simulink model "sampleModel27"  (R2021b)
settings: Solver=VariableStepAuto  StartTime=0.0  StopTime=10.0  RelTol=1e-3
undefined symbols (not defined in the file or in its folder): Newton, Raphson
libraries: simulink x5, slpidlib x1
settings Model: Creator=user  LastModifiedBy=user

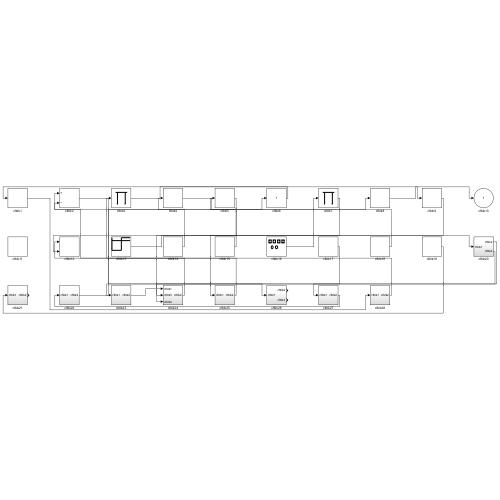
[thumbnail: Simulink's stored preview of the top-level diagram]
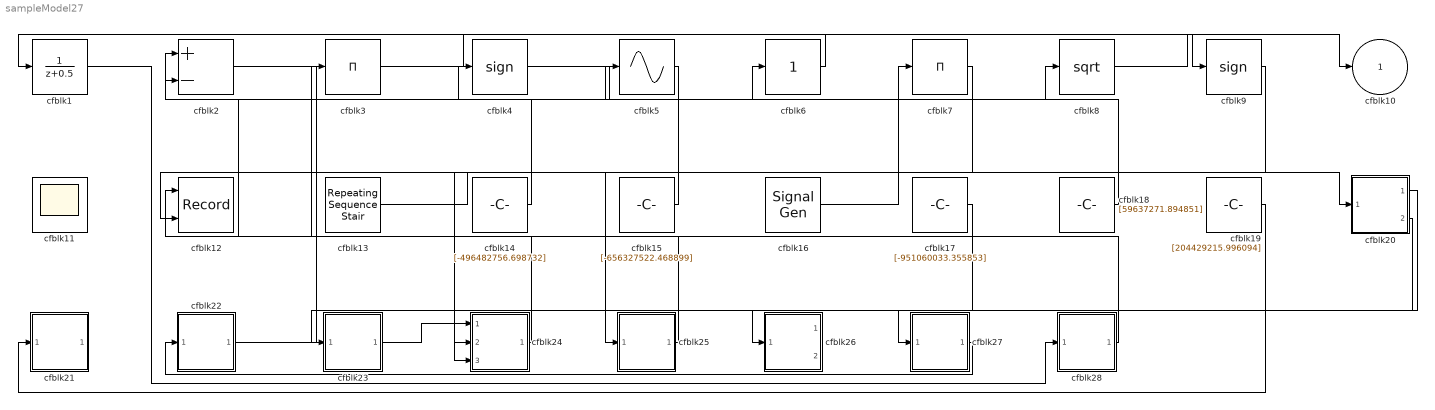
== system sampleModel27 ==
  cfblk1 : DiscreteTransferFcn  SampleTime=1
  cfblk11 : Scope
      settings: Floating=on
  cfblk12 : Record  FileSettingsInternal="{\"entries\":[{\"content\":{\"excelSettings\":{\"content\":{},\"type\":\"Streamout.ExcelSettings\"}},\"type\":\"Streamout.FileSettingStorage\",\"uuid\":\"817101b1-7ee6-489f-8bf2-f4af326754e9\"}],\"packageUris\":[\"http://schema.mathworks.com/mf0/streamout_blocks/R2020a\"],\"version\":\"1.0\"}"  Layout=[1 1]  SignalsInternal="{\"entries\":[{\"content\":{\"signals\":[{\"content\":{\"blockPath\":[\"sampleModel27/cfblk12\"],\"channel\":[],\"dimensions\":[1],\"domain\":\"sampleModel27/cfblk12\",\"lineColor\":\"#a2142f\",\"plots\":[1],\"port\":1,\"sid\":[\"\"],\"signalID\":1067,\"signalName\":\"cfblk24\"},\"type\":\"RecordBlkView.Signal\",\"uuid\":\"11552be4-8ecd-494b-946a-d208da3a0090\"},{\"content\":{\"blockPath\":[\"sampleModel27/cfblk12\"],\"channel\":[],\"dimensions\":[1],\"domain\":\"sampleModel27/cfblk12\",\"lineColor\":\"#139fff\",\"plots\":[1],\"port\":2,\"sid\":[\"\"],\"signalID\":1071,\"signalName\":\"cfblk9\"},\"type\":\"RecordBlkView.Signal\",\"uuid\":\"e2f3f9ab-da11-493e-9bea-993bb7e61e53\"}]},\"type\":\"RecordBlkView.InputSignals\",\"uuid\":\"027c9f95-9f0f-4801-a41c-29daeef56658\"}],\"packageUris\":[\"http://schema.mathworks.com/mf0/streamout_blocks/R2020a\"],\"version\":\"1.0\"}"  VisualizationBindings="{\"xyplotplugin\":{\"info\":[{\"series\":[{\"bindingParametersList\":[{\"parameter\":\"X-Axis\",\"signalID\":1067,\"signalName\":\"cfblk24\"},{\"parameter\":\"Y-Axis\",\"signalID\":1071,\"signalName\":\"cfblk9\"}],\"seriesID\":40632}],\"subplotID\":1}]}}"  CompatibilityTag=XY
  cfblk13 : simulink/Sources/Repeating Sequence Stair  OutValues=[-914274327.688707, 278326402.924223]  tsamp=-1  OutMin=[]  OutMax=[]  OutDataTypeStr=double  OutputDataTypeScalingMode=double  OutDataType=fixdt(0,8)  ConRadixGroup=Best Precision: Vector-wise  OutScaling=2^-12
  cfblk14 : Constant  Value=[-496482756.698732]  SampleTime=1
  cfblk15 : Constant  Value=[-656327522.468899]  SampleTime=1
  cfblk16 : SignalGenerator  Amplitude=[-317971779.391681]
  cfblk17 : Constant  Value=[-951060033.355853]  SampleTime=1
  cfblk18 : Constant  Value=[59637271.894851]  SampleTime=1
  cfblk19 : Constant  Value=[204429215.996094]  SampleTime=1
  cfblk2 : Sum  Inputs=+-
  cfblk20 : Subsystem
  cfblk21 : Subsystem
  cfblk22 : Subsystem
  cfblk23 : Subsystem
  cfblk24 : Subsystem
  cfblk25 : Subsystem
  cfblk26 : Subsystem
  cfblk27 : Subsystem
  cfblk28 : Subsystem
  cfblk3 : Product  Inputs=*
  cfblk4 : Signum
  cfblk5 : Sin  TimeSource=Use external signal  SampleTime=0
  cfblk6 : simulink/Math Operations/Slider Gain  gain=1  low=0  high=2
  cfblk7 : Product  Inputs=*
  cfblk8 : Sqrt  SaturateOnIntegerOverflow=on
  cfblk9 : Signum
  cfblk10 : Outport
  wires:
  cfblk3/1 -> cfblk9/1
  cfblk7/1 -> cfblk25/1(cfblk1)
  cfblk24/1(cfblk2) -> cfblk12/1
  cfblk9/1 -> cfblk12/2
  cfblk2/1 -> cfblk26/1(cfblk1)
  cfblk27/1(cfblk2) -> cfblk22/1(cfblk1)
  cfblk16/1 -> cfblk7/1
  cfblk28/1(cfblk2) -> cfblk3/1
  cfblk17/1 -> cfblk27/1(cfblk1)
  cfblk4/1 -> cfblk6/1
  cfblk1/1 -> cfblk28/1(cfblk1)
  cfblk14/1 -> cfblk2/1
  cfblk6/1 -> cfblk1/1
  cfblk19/1 -> cfblk21/1(cfblk1)
  cfblk15/1 -> cfblk5/1
  cfblk8/1 -> cfblk10/1
  cfblk18/1 -> cfblk4/1
  cfblk23/1(cfblk2) -> cfblk24/1(cfblk1)
  cfblk22/1(cfblk2) -> cfblk8/1
  cfblk13/1 -> cfblk20/1(cfblk1)
  cfblk25/1(cfblk2) -> cfblk2/2
  cfblk5/1 -> cfblk24/2(cfblk3)
  cfblk20/1(cfblk2) -> cfblk23/1(cfblk1)
  cfblk20/2(cfblk4) -> cfblk24/3(cfblk4)

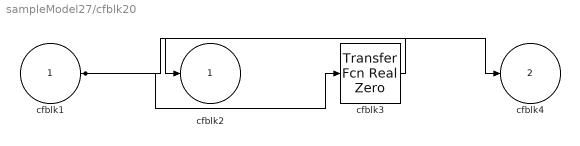
== system sampleModel27/cfblk20 ==
  cfblk1 : Inport
  cfblk3 : simulink/Discrete/Transfer Fcn Real Zero  ZeroZ=0.75  ICPrevInput=0.0  DoSatur=off
      settings: SourceProductBaseCode=SL
  cfblk2 : Outport
  cfblk4 : Outport  Port=2
  wires:
  cfblk3/1 -> cfblk2/1
  cfblk1/1 -> cfblk3/1, cfblk4/1

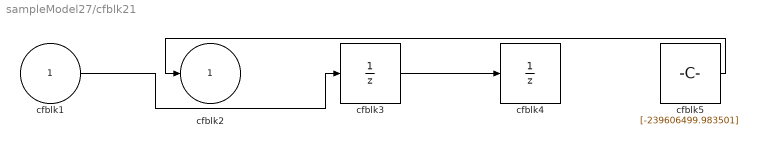
== system sampleModel27/cfblk21 ==
  cfblk1 : Inport
  cfblk3 : UnitDelay  HasFrameUpgradeWarning=on
  cfblk4 : UnitDelay  HasFrameUpgradeWarning=on
  cfblk5 : Constant  Value=[-239606499.983501]  SampleTime=1
  cfblk2 : Outport
  wires:
  cfblk5/1 -> cfblk2/1
  cfblk3/1 -> cfblk4/1
  cfblk1/1 -> cfblk3/1

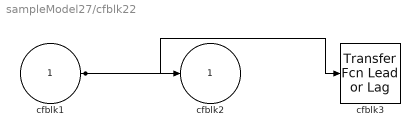
== system sampleModel27/cfblk22 ==
  cfblk1 : Inport
  cfblk3 : simulink/Discrete/Transfer Fcn Lead or Lag  PoleZ=0.95  ZeroZ=0.75  ICPrevOutput=0.0  ICPrevInput=0.0  DoSatur=off
      settings: SourceProductBaseCode=SL
  cfblk2 : Outport
  wires:
  cfblk1/1 -> cfblk2/1, cfblk3/1

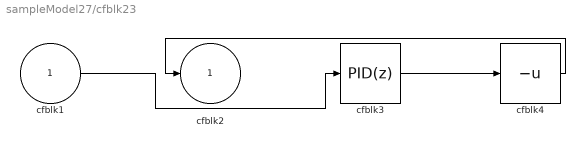
== system sampleModel27/cfblk23 ==
  cfblk1 : Inport
  cfblk3 : slpidlib/PID Controller  Controller=PID  Form=Parallel  TimeDomain=Discrete-time  UseExternalTs=off  SampleTime=1  IntegratorMethod=Forward Euler  FilterMethod=Forward Euler  ControllerParametersSource=internal  P=1  I=1  D=0  UseFilter=on  N=100  TunerSelectOption=Transfer Function Based (PID Tuner App)  InitialConditionSource=internal  InitialConditionForIntegrator=0  InitialConditionForFilter=0  DifferentiatorICPrevScaledInput=0  ExternalReset=none  TrackingMode=off  Kt=1  LimitOutput=off  SatLimitsSource=internal  UpperSaturationLimit=inf  LowerSaturationLimit=-inf  LinearizeAsGain=off  AntiWindupMode=none  Kb=1  POutMin=[]  POutMax=[]  IOutMin=[]  IOutMax=[]  DOutMin=[]  DOutMax=[]  NOutMin=[]  NOutMax=[]  SumOutMin=[]  SumOutMax=[]  SaturationOutMin=[]  SaturationOutMax=[]  PParamMin=[]  PParamMax=[]  IParamMin=[]  IParamMax=[]  DParamMin=[]  DParamMax=[]  NParamMin=[]  NParamMax=[]  KbParamMin=[]  KbParamMax=[]  KtParamMin=[]  KtParamMax=[]  KbOutMin=[]  KbOutMax=[]  KtOutMin=[]  KtOutMax=[]  IntegratorOutMin=[]  IntegratorOutMax=[]  FilterOutMin=[]  FilterOutMax=[]  SumI1OutMin=[]  SumI1OutMax=[]  SumI2OutMin=[]  SumI2OutMax=[]  SumI3OutMin=[]  SumI3OutMax=[]  SumI4OutMin=[]  SumI4OutMax=[]  SumDOutMin=[]  SumDOutMax=[]  DifferentiatorOutMin=[]  DifferentiatorOutMax=[]  FilterDiffOutCoefMin=[]  FilterDiffOutCoefMax=[]  ReciprocalOutMin=[]  ReciprocalOutMax=[]  SumDenOutMin=[]  SumDenOutMax=[]  SumNumOutMin=[]  SumNumOutMax=[]  DivideOutMin=[]  DivideOutMax=[]  UdiffTsProdOutMin=[]  UdiffTsProdOutMax=[]  NTsProdOutMin=[]  NTsProdOutMax=[]  UintegralTsProdOutMin=[]  UintegralTsProdOutMax=[]  UngainTsProdOutMin=[]  UngainTsProdOutMax=[]  IntegratorContinuousStateAttributes=''  IntegratorStateMustResolveToSignalObject=off  IntegratorRTWStateStorageClass=Auto  FilterContinuousStateAttributes=''  FilterStateMustResolveToSignalObject=off  FilterRTWStateStorageClass=Auto  ParallelPVariant=InternalParameters  IdealPVariant=Disabled  IVariant=InternalParameters  DVariant=InternalParameters  IntegratorVariant=Discrete  SatVariant=Disabled  AWVariant=Passthrough  PCopyVariant=Disabled  TRVariant=Disabled  FdbkBlocksVariant=Forward  IdealPFdbkVariant=Disabled  SatFdbkVariant=Disabled  DerivativeFilterVariant=ForwardEulerFilter  NVariant=InternalParameters  NCopyVariant=Disabled  FilterICVariant=InternalICsFilter  IntegratorICVariant=InternalICs  ExternalResetVariant=Disabled  TRSumVariant=Passthrough  SumFdbkVariant=Disabled  SumVariant=Sum_PID  TsampFilterVariant=InternalTs  TsampNgainVariant=Passthrough  TsampIntegralVariant=Passthrough  ExternalSaturationOutDataTypeStr=Inherit: Same as second input
  cfblk4 : UnaryMinus
  cfblk2 : Outport
  wires:
  cfblk4/1 -> cfblk2/1
  cfblk1/1 -> cfblk3/1
  cfblk3/1 -> cfblk4/1

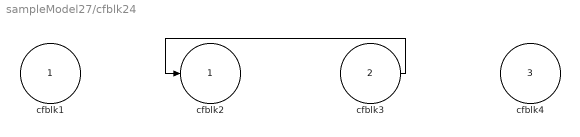
== system sampleModel27/cfblk24 ==
  cfblk1 : Inport
  cfblk3 : Inport  Port=2
  cfblk4 : Inport  Port=3
  cfblk2 : Outport
  wires:
  cfblk3/1 -> cfblk2/1

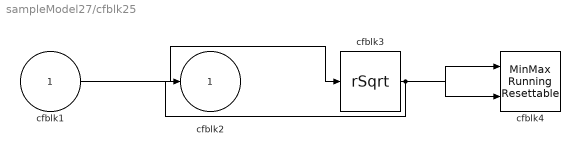
== system sampleModel27/cfblk25 ==
  cfblk1 : Inport
  cfblk3 : Sqrt  Operator=rSqrt  AlgorithmType=Newton-Raphson  SaturateOnIntegerOverflow=on
  cfblk4 : simulink/Math Operations/MinMax Running Resettable  Function=min  vinit=0.0
  cfblk2 : Outport
  wires:
  cfblk1/1 -> cfblk3/1
  cfblk3/1 -> cfblk2/1, cfblk4/1, cfblk4/2

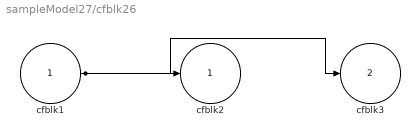
== system sampleModel27/cfblk26 ==
  cfblk1 : Inport
  cfblk2 : Outport
  cfblk3 : Outport  Port=2
  wires:
  cfblk1/1 -> cfblk3/1, cfblk2/1

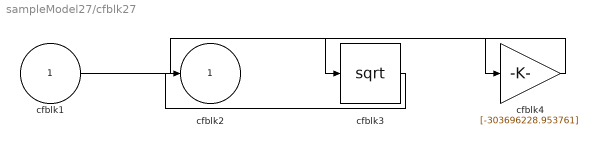
== system sampleModel27/cfblk27 ==
  cfblk1 : Inport
  cfblk3 : Sqrt  SaturateOnIntegerOverflow=on
  cfblk4 : Gain  Gain=[-303696228.953761]
  cfblk2 : Outport
  wires:
  cfblk1/1 -> cfblk4/1
  cfblk3/1 -> cfblk2/1
  cfblk4/1 -> cfblk3/1

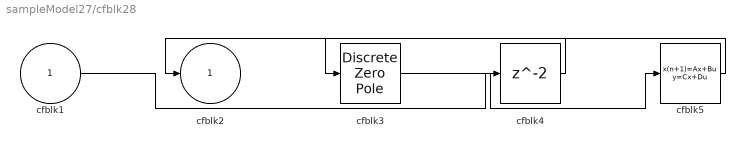
== system sampleModel27/cfblk28 ==
  cfblk1 : Inport
  cfblk3 : DiscreteZeroPole  Poles=[0 0.5]  Gain=1
  cfblk4 : Delay  SampleTime=1
  cfblk5 : DiscreteStateSpace
  cfblk2 : Outport
  wires:
  cfblk5/1 -> cfblk2/1
  cfblk3/1 -> cfblk5/1
  cfblk4/1 -> cfblk3/1
  cfblk1/1 -> cfblk4/1
